simulink model "Estimation_of_Rint_Model_Parameters"  (R2021a)
settings: Solver=VariableStepAuto  StartTime=0.0  StopTime=3600  RelTol=1e-3
values from neighbouring files (symbols this model uses):
  A_cell = cell_length*cell_width    (= 0.051302)    [RintModel_Script.m]
  Capacity = 31.000    (= 31)    [RintModel_Script.m]
  Cp_cell = 810.5328    [RintModel_Script.m]
  H_cell = 5    [RintModel_Script.m]
  M_cell = 0.72    [RintModel_Script.m]
  OCV_LUT = [3.49; 3.55; 3.62; 3.71; 3.91; 4.17; 4.19]    [RintModel_Script.m]
  R_int_LUT = [0.0085; 0.0085; 0.0087; 0.0082; 0.0083; 0.0085; 0.0085]    [RintModel_Script.m]
  SOC_LUT = [0; 0.1; 0.25; 0.5; 0.75; 0.9; 1.0]    [RintModel_Script.m]
  T_amb = 293.15    [RintModel_Script.m]
libraries: simulink x1
settings Model: Creator=gopin  LastModifiedBy=gopin

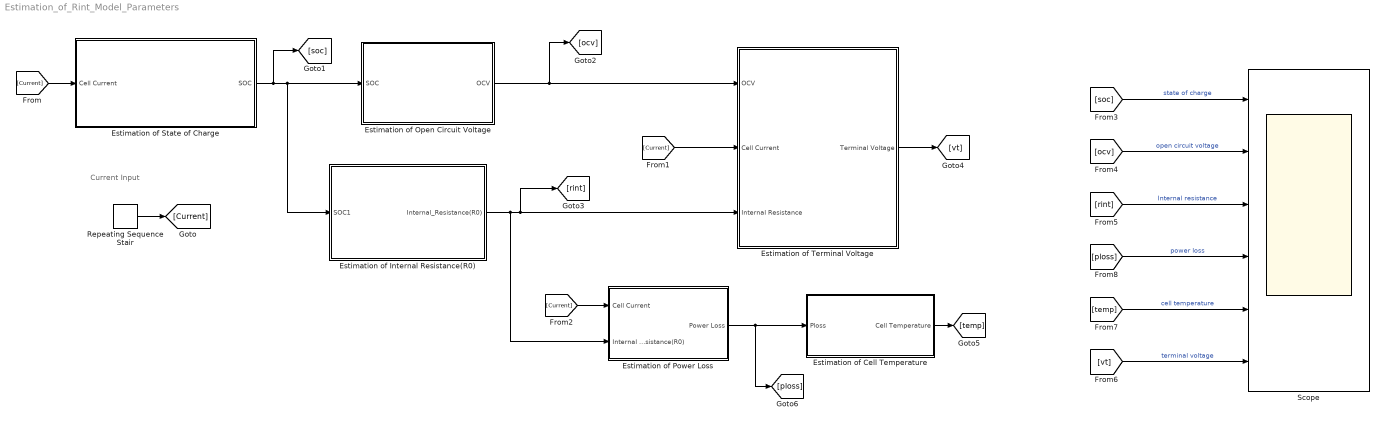
== system Estimation_of_Rint_Model_Parameters ==
  note: Current Input
  Estimation of Cell Temperature : Subsystem
  Estimation of Internal Resistance(R0) : Subsystem
  Estimation of Open Circuit Voltage : Subsystem
  Estimation of Power Loss : Subsystem
  "Estimation of State of Charge " : Subsystem
  Estimation of Terminal Voltage : Subsystem
  Repeating Sequence Stair : simulink/Sources/Repeating Sequence Stair  OutValues=[0 0 0 5 9 15 18 18 18 11 8 3 1]  tsamp=-1  OutMin=[]  OutMax=[]  OutDataTypeStr=double  OutputDataTypeScalingMode=double  OutDataType=fixdt(0,8)  ConRadixGroup=Best Precision: Vector-wise  OutScaling=2^-12
  Scope : Scope  NumInputPorts=6
  wires:
  "Estimation of State of Charge "/1(SOC) -> [soc], Estimation of Internal Resistance(R0)/1(SOC1), Estimation of Open Circuit Voltage/1(SOC)
  Estimation of Open Circuit Voltage/1(OCV) -> [ocv], Estimation of Terminal Voltage/1(OCV)
  Estimation of Internal Resistance(R0)/1(Internal_Resistance(R0)) -> [rint], Estimation of Terminal Voltage/3(Internal Resistance), Estimation of Power Loss/2(Internal Resistance(R0))
  Estimation of Power Loss/1(Power Loss) -> [ploss], Estimation of Cell Temperature/1(Ploss)
  Repeating Sequence Stair/1 -> [Current]
  [Current] -> "Estimation of State of Charge "/1(Cell Current)
  [Current] -> Estimation of Terminal Voltage/2(Cell Current)
  [Current] -> Estimation of Power Loss/1(Cell Current)
  Estimation of Cell Temperature/1(Cell Temperature) -> [temp]
  Estimation of Terminal Voltage/1(Terminal Voltage) -> [vt]
  [soc] -> Scope/1  "state of charge"
  [ocv] -> Scope/2  "open circuit voltage"
  [vt] -> Scope/6  "terminal voltage"
  [temp] -> Scope/5  "cell temperature"
  [ploss] -> Scope/4  "power loss"
  [rint] -> Scope/3  "Internal resistance"

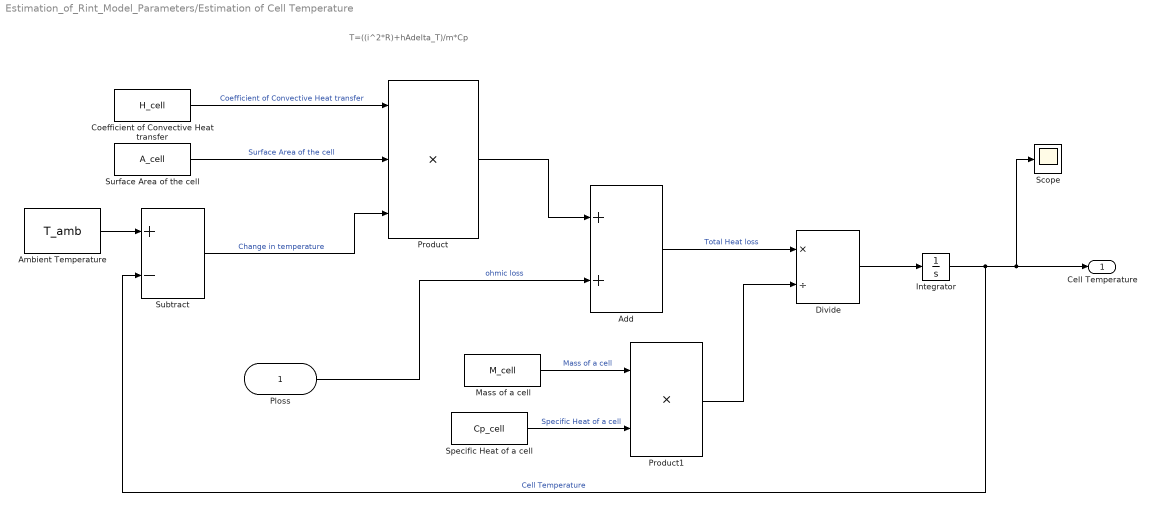
== system Estimation_of_Rint_Model_Parameters/Estimation of Cell Temperature ==
  note: T=((i^2*R)+hAdelta_T)/m*Cp
  Ploss : Inport
  Add : Sum
  Ambient Temperature : Constant  Value=T_amb
  Coefficient of Convective Heat transfer : Constant  Value=H_cell
  Divide : Product  Inputs=*/
  Integrator : Integrator  InitialCondition=T_amb
  Mass of a cell : Constant  Value=M_cell
  Product : Product  Inputs=3
  Product1 : Product
  Scope : Scope
  Specific Heat of a cell : Constant  Value=Cp_cell
  Subtract : Sum  Inputs=+-
  Surface Area of the cell : Constant  Value=A_cell
  Cell Temperature : Outport
  wires:
  Ambient Temperature/1 -> Subtract/1
  Coefficient of Convective Heat transfer/1 -> Product/1  "Coefficient of Convective Heat transfer"
  Surface Area of the cell/1 -> Product/2  "Surface Area of the cell"
  Subtract/1 -> Product/3  "Change in temperature"
  Product/1 -> Add/1
  Ploss/1 -> Add/2  "ohmic loss"
  Add/1 -> Divide/1  "Total Heat loss"
  Product1/1 -> Divide/2
  Mass of a cell/1 -> Product1/1  "Mass of a cell"
  Specific Heat of a cell/1 -> Product1/2  "Specific Heat of a cell"
  Divide/1 -> Integrator/1
  Integrator/1 -> Subtract/2, Scope/1, Cell Temperature/1  "Cell Temperature"

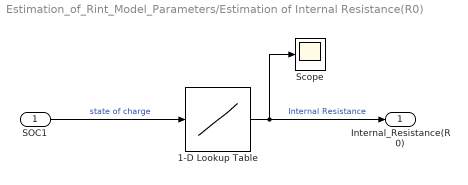
== system Estimation_of_Rint_Model_Parameters/Estimation of Internal Resistance(R0) ==
  SOC1 : Inport
  1-D Lookup Table : Lookup_n-D  NumberOfTableDimensions=1  BreakpointsForDimension1=SOC_LUT  Table=R_int_LUT  InternalRulePriority=Speed  RndMeth=Simplest  InputSameDT=on
  Scope : Scope
  Internal_Resistance(R0) : Outport
  wires:
  SOC1/1 -> 1-D Lookup Table/1  "state of charge"
  1-D Lookup Table/1 -> Scope/1, Internal_Resistance(R0)/1  "Internal Resistance"

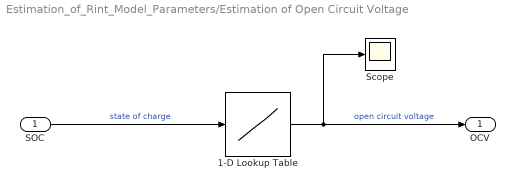
== system Estimation_of_Rint_Model_Parameters/Estimation of Open Circuit Voltage ==
  SOC : Inport
  1-D Lookup Table : Lookup_n-D  NumberOfTableDimensions=1  BreakpointsForDimension1=SOC_LUT  Table=OCV_LUT  InternalRulePriority=Speed  RndMeth=Simplest  InputSameDT=on
  Scope : Scope
  OCV : Outport
  wires:
  SOC/1 -> 1-D Lookup Table/1  "state of charge"
  1-D Lookup Table/1 -> Scope/1, OCV/1  "open circuit voltage"

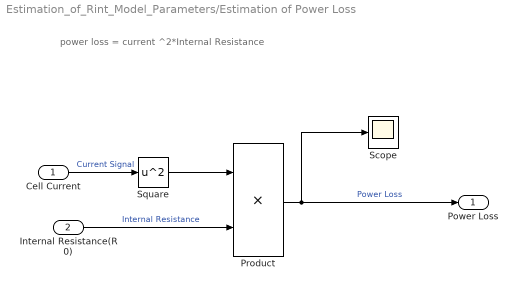
== system Estimation_of_Rint_Model_Parameters/Estimation of Power Loss ==
  note: power loss = current ^2*Internal Resistance
  Cell Current : Inport
  Internal Resistance(R0) : Inport  Port=2
  Product : Product
  Scope : Scope
  Square : Math  Operator=square  SaturateOnIntegerOverflow=on
  Power Loss : Outport
  wires:
  Cell Current/1 -> Square/1  "Current Signal"
  Square/1 -> Product/1
  Product/1 -> Scope/1, Power Loss/1  "Power Loss"
  Internal Resistance(R0)/1 -> Product/2  "Internal Resistance"

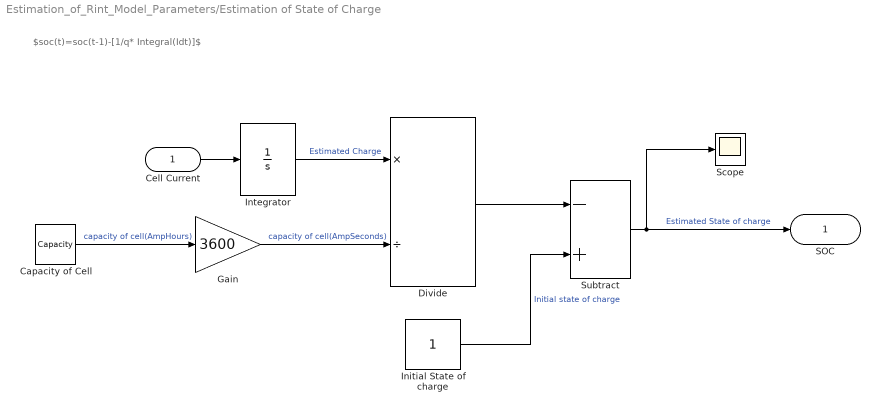
== system Estimation_of_Rint_Model_Parameters/Estimation of State of Charge  ==
  note: $soc(t)=soc(t-1)-[1/q* Integral(Idt)]$
  Cell Current : Inport
  Capacity of Cell : Constant  Value=Capacity
  Divide : Product  Inputs=*/
  Gain : Gain  Gain=3600
  Initial State of charge : Constant
  Integrator : Integrator
  Scope : Scope
  Subtract : Sum  Inputs=-+
  SOC : Outport
  wires:
  Initial State of charge/1 -> Subtract/2  "Initial state of charge"
  Subtract/1 -> Scope/1, SOC/1  "Estimated State of charge"
  Integrator/1 -> Divide/1  "Estimated Charge"
  Divide/1 -> Subtract/1
  Cell Current/1 -> Integrator/1
  Capacity of Cell/1 -> Gain/1  "capacity of cell(AmpHours)"
  Gain/1 -> Divide/2  "capacity of cell(AmpSeconds)"

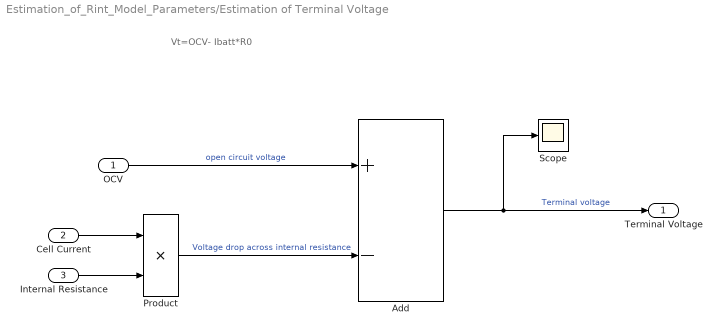
== system Estimation_of_Rint_Model_Parameters/Estimation of Terminal Voltage ==
  note: Vt=OCV- Ibatt*R0
  OCV : Inport
  Cell Current : Inport  Port=2
  Internal Resistance : Inport  Port=3
  Add : Sum  Inputs=+-
  Product : Product
  Scope : Scope
  Terminal Voltage : Outport
  wires:
  Add/1 -> Scope/1, Terminal Voltage/1  "Terminal voltage"
  OCV/1 -> Add/1  "open circuit voltage"
  Product/1 -> Add/2  "Voltage drop across internal resistance"
  Cell Current/1 -> Product/1
  Internal Resistance/1 -> Product/2
